simulink model "VB_RI_EKF_GNSS_INS25"  (R2023a)
settings: Solver=FixedStepAuto  StartTime=0  StopTime=200  FixedStep=0.01  RelTol=1e-3
InitFcn:
  | %resilient_initNavigation1216;
  | %init_param;
values from neighbouring files (symbols this model uses):
  C = zeros(n,m)    [utchol.m]
undefined symbols (not defined in the file or in its folder): dt, dtDelay, g0, gam0_rad, GNSSoutragetime, ISUS_flag, magnitude, p, P0, P0_RIEKF, param, pd0, pe0, phi0_rad, pn0, psi, psi0_rad, state_dim, vd0, ve0, vn0
libraries: simulink_extras x133, simulink x81, dspstat3 x81, sharedtransform x69, sharedTrackingLibrary x17, matrix_library x15, deeplib x6, dspfactors x4, aerolibconvert2 x4, aerolibtransform2 x4, dspsrcs4 x1
(part 13 of 32)

== system VB_RI_EKF_GNSS_INS25/ISUS_RIEKF3/Error State Kalman Filter M1/VB-Extended Kalman Filter M2 ==
  Q : Inport
  Enable1 : Inport  Port=2
  y1 : Inport  Port=3
  R1 : Inport  Port=4
  H : Inport  Port=5
  pk_1 : Inport  Port=6
  pk_2 : Inport  Port=7
  BlockOrdering : Constant  Value=true()  OutDataTypeStr=boolean
  Correct M1 : Subsystem  AncestorBlock=sharedTrackingLibrary/Extras/EKFCorrect  TreatAsAtomicUnit=on  SystemSampleTime=p.SampleTimes.MeasurementFcn(1)  mask(EKFCorrect){ProcessedMaskData=p}
      mask init: same as VB_RI_EKF_GNSS_INS25/ER EKF/Error State Kalman Filter/Extended Kalman Filter1/Correct1
      settings: LibrarySourceBlock=sharedTrackingLibrary/Extras/EKFCorrect
  Data Store Read : DataStoreRead  Commented=on  DataStoreName=P  IndexOptions=Index vector (dialog)  Indices=1  OutputSizes=1
  Data Store Read1 : DataStoreRead  Commented=on  DataStoreName=x  IndexOptions=Index vector (dialog)  Indices=1  OutputSizes=1
  DataStoreMemory - P : DataStoreMemory  DataStoreName=P  InitialValue=p.InitialCovariance  ShowAdditionalParam=off  OutDataTypeStr=p.DataType
  DataStoreMemory - x : DataStoreMemory  DataStoreName=x  InitialValue=p.InitialState  ShowAdditionalParam=off  OutDataTypeStr=p.DataType
  DataTypeConversion_Enable1 : DataTypeConversion  OutDataTypeStr=boolean  SaturateOnIntegerOverflow=off  RndMeth=Floor
  DataTypeConversion_Q : DataTypeConversion  OutDataTypeStr=p.DataType  SaturateOnIntegerOverflow=off  RndMeth=Floor
  DataTypeConversion_R1 : DataTypeConversion  OutDataTypeStr=p.DataType  SaturateOnIntegerOverflow=off  RndMeth=Floor
  DataTypeConversion_uMeas1 : DataTypeConversion  OutDataTypeStr=p.DataType  SaturateOnIntegerOverflow=off  RndMeth=Floor
  DataTypeConversion_uState : DataTypeConversion  OutDataTypeStr=p.DataType  SaturateOnIntegerOverflow=off  RndMeth=Floor
  DataTypeConversion_y1 : DataTypeConversion  OutDataTypeStr=p.DataType  SaturateOnIntegerOverflow=off  RndMeth=Floor
  MeasurementFcn1Inputs : Constant  Value=0  OutDataTypeStr=p.DataType  SampleTime=p.SampleTimes.MeasurementFcn(1)
  Output : Subsystem  TreatAsAtomicUnit=on  SystemSampleTime=p.SampleTimes.Output
  Predict : Subsystem  TreatAsAtomicUnit=on  SystemSampleTime=p.SampleTimes.StateTransitionFcn  mask(EKFPredict){ProcessedMaskData=p}
      mask init: same as VB_RI_EKF_GNSS_INS25/ER EKF/Error State Kalman Filter/Extended Kalman Filter1/Predict
  StateTransitionFcnInputs : Constant  Value=0  OutDataTypeStr=p.DataType  SampleTime=p.SampleTimes.StateTransitionFcn
  checkMeasurementFcn1Signals : S-Function  FunctionName=ekfukfCheckSignals  Parameters=signalCheck.BlockPath, signalCheck.MeasurementFcn{1}.PortNames, signalCheck.MeasurementFcn{1}.SampleTime, signalCheck.DataType, signalCheck.MeasurementFcn{1}.PortDimensions, 1, signalCheck.MeasurementFcn{1}.HasAdditiveNoise  SFunctionDeploymentMode=off  EnableBusSupport=off
  checkStateTransitionFcnSignals : S-Function  FunctionName=ekfukfCheckSignals  Parameters=signalCheck.BlockPath, signalCheck.StateTransitionFcn.PortNames, signalCheck.StateTransitionFcn.SampleTime, signalCheck.DataType, signalCheck.StateTransitionFcn.PortDimensions, 0, signalCheck.StateTransitionFcn.HasAdditiveNoise  SFunctionDeploymentMode=off  EnableBusSupport=off
  innovation calculation : Subsystem  Commented=on
  xhat : Outport  VectorParamsAs1DForOutWhenUnconnected=off
  P : Outport  Port=2
  Sk : Outport  Port=3  VectorParamsAs1DForOutWhenUnconnected=off
  m_innov : Outport  Port=4  VectorParamsAs1DForOutWhenUnconnected=off
  wires:
  [AfterOutput] -> Predict/3(uBlockOrdering)
  Output/3(yBlockOrdering) -> [AfterOutput]
  [AfterCorrect] -> Output/1(uBlockOrdering)
  [FirstOperation] -> Correct M1/4(uBlockOrdering)
  BlockOrdering/1 -> [FirstOperation]
  DataTypeConversion_uMeas1/1 -> Correct M1/3(uMeas)
  DataTypeConversion_R1/1 -> Correct M1/2(R), innovation calculation/4(R)
  MeasurementFcn1Inputs/1 -> DataTypeConversion_uMeas1/1, checkMeasurementFcn1Signals/4
  DataTypeConversion_y1/1 -> innovation calculation/2(yMeas), Correct M1/1(yMeas)
  DataTypeConversion_uState/1 -> Predict/2(uState)
  StateTransitionFcnInputs/1 -> DataTypeConversion_uState/1, checkStateTransitionFcnSignals/2
  DataTypeConversion_Enable1/1 -> Correct M1/Enable
  Enable1/1 -> DataTypeConversion_Enable1/1, checkMeasurementFcn1Signals/1
  DataTypeConversion_Q/1 -> Predict/1(Q)
  Q/1 -> DataTypeConversion_Q/1, checkStateTransitionFcnSignals/1
  R1/1 -> DataTypeConversion_R1/1, checkMeasurementFcn1Signals/3
  y1/1 -> DataTypeConversion_y1/1, checkMeasurementFcn1Signals/2
  Output/1(x) -> xhat/1
  Correct M1/1(yBlockOrdering) -> [AfterCorrect]
  H/1 -> innovation calculation/5(H), Correct M1/5(H)
  pk_1/1 -> Correct M1/6(pk_1)
  Output/2(P) -> P/1
  Data Store Read/1 -> innovation calculation/1(Pk/k_1)
  Data Store Read1/1 -> innovation calculation/3(X)
  Correct M1/2(Sk) -> Sk/1
  Correct M1/3(m_innov) -> m_innov/1
  pk_2/1 -> Correct M1/7(P)

== system VB_RI_EKF_GNSS_INS25/ISUS_RIEKF3/Error State Kalman Filter M1/bak ==
  From1 : From  Commented=on  GotoTag=wxyz
  From11 : From  Commented=on  GotoTag=p_INS
  From14 : From  Commented=on  GotoTag=DCM_b_n
  From2 : From  Commented=on  GotoTag=fbxyz
  From3 : From  Commented=on  GotoTag=ZUPTenable
  From4 : From  Commented=on  GotoTag=v_INS
  From5 : From  Commented=on  GotoTag=fex
  From6 : From  Commented=on  GotoTag=DCM_b_n
  From9 : From  Commented=on  GotoTag=DCM_b_n
  Goto6 : Goto  Commented=on  GotoTag=ZUPTenable
  MATLAB Function1 : MATLAB Function  Commented=on  TreatAsAtomicUnit=on
  Memory1 : Memory  Commented=on
  RIEKF : MATLAB Function  Commented=on  TreatAsAtomicUnit=on
  Rate Transition2 : RateTransition  Commented=on  OutPortSampleTime=dt
  Scope10 : Scope  Commented=on  NumInputPorts=2
  Simulink Function - GPS Measurements1 : Subsystem  Commented=on  TreatAsAtomicUnit=on
  Simulink Function - GPS Measurements2 : Subsystem  Commented=on  TreatAsAtomicUnit=on
  Simulink Function - State Transition Jacobian : Subsystem  Commented=on  TreatAsAtomicUnit=on
  Unscented Kalman Filter1 : sharedTrackingLibrary/Unscented Kalman Filter  Commented=on  StateTransitionFcn=stateTransitionFcn_Dyn  HasAdditiveProcessNoise=Nonadditive  ProcessNoise=1  HasTimeVaryingProcessNoise=on  HasStateTransitionFcnExtraArgument=0  InitialState=zeros(18,1)  InitialStateCovariance=diag([1*ones(3,1);0.1*ones(3,1);0.001*ones(3,1);0.001*ones(6,1);0.1*ones(3,1)]);  Alpha=1e-2  Beta=2  Kappa=0  MeasurementFcn1=GPSMeasurementFcn_Dyn  HasMeasurementEnablePort1=on  HasAdditiveMeasurementNoise1=Nonadditive  MeasurementNoise1=1  HasTimeVaryingMeasurementNoise1=on  HasMeasurementFcnExtraArgument1=0  HasMeasurementWrapping1=off  MeasurementFcn2=DynamicMeasurementFcn_Dyn  HasMeasurementEnablePort2=on  HasAdditiveMeasurementNoise2=Nonadditive  MeasurementNoise2=1  HasTimeVaryingMeasurementNoise2=on  HasMeasurementFcnExtraArgument2=0  HasMeasurementWrapping2=off  MeasurementFcn3=myMeasurementFcn  HasMeasurementEnablePort3=off  HasAdditiveMeasurementNoise3=Additive  MeasurementNoise3=1  HasTimeVaryingMeasurementNoise3=off  HasMeasurementFcnExtraArgument3=0  HasMeasurementWrapping3=off  MeasurementFcn4=myMeasurementFcn  HasMeasurementEnablePort4=off  HasAdditiveMeasurementNoise4=Additive  MeasurementNoise4=1  HasTimeVaryingMeasurementNoise4=off  HasMeasurementFcnExtraArgument4=0  HasMeasurementWrapping4=off  MeasurementFcn5=myMeasurementFcn  HasMeasurementEnablePort5=off  HasAdditiveMeasurementNoise5=Additive  MeasurementNoise5=1  HasTimeVaryingMeasurementNoise5=off  HasMeasurementFcnExtraArgument5=0  HasMeasurementWrapping5=off  EnableMultirate=off  StateTransitionFcnSampleTime=1  MeasurementFcn1SampleTime=1  MeasurementFcn2SampleTime=1  MeasurementFcn3SampleTime=1  MeasurementFcn4SampleTime=1  MeasurementFcn5SampleTime=1  UseCurrentEstimator=on  OutputStateCovariance=on  DataType=single  SampleTime=0.01  NumberOfMeasurements=2
  Out1 : Outport
  wires:
  From14/1 -> Simulink Function - GPS Measurements1/1(DCM_b_n)
  From4/1 -> Simulink Function - State Transition Jacobian/2(vn)
  From9/1 -> Simulink Function - State Transition Jacobian/1(DCM_b_n)
  From11/1 -> Simulink Function - State Transition Jacobian/3(pn)
  From3/1 -> Rate Transition2/1
  MATLAB Function1/2(ZeroVelDetectFlagold) -> Scope10/2
  From6/1 -> MATLAB Function1/1(Cbn)
  From2/1 -> MATLAB Function1/3(fbxyz)
  From5/1 -> Memory1/1
  MATLAB Function1/1(ZeroVelDetectFlag) -> Goto6/1, Scope10/1
  From1/1 -> MATLAB Function1/2(wxyz)
  Rate Transition2/1 -> Out1/1
  Memory1/1 -> MATLAB Function1/4(fex)

== system VB_RI_EKF_GNSS_INS25/ISUS_RIEKF3/Error State Kalman Filter M2/Cal Q1 ==
  Constant : Constant  Value=dt  OutDataTypeStr=double
  MATLAB Function1 : MATLAB Function  TreatAsAtomicUnit=on
  Qd : Outport
  wires:
  Constant/1 -> MATLAB Function1/1(dt)
  MATLAB Function1/1(Q) -> Qd/1

== system VB_RI_EKF_GNSS_INS25/ISUS_RIEKF3/Error State Kalman Filter M2/Extended Kalman Filter M1 ==
  Q : Inport
  Enable1 : Inport  Port=2
  y1 : Inport  Port=3
  R1 : Inport  Port=4
  H : Inport  Port=5
  pk_1 : Inport  Port=6
  beta_2 : Inport  Port=7
  BlockOrdering : Constant  Value=true()  OutDataTypeStr=boolean
  Correct M1 : Subsystem  AncestorBlock=sharedTrackingLibrary/Extras/EKFCorrect  TreatAsAtomicUnit=on  SystemSampleTime=p.SampleTimes.MeasurementFcn(1)  mask(EKFCorrect){ProcessedMaskData=p}
      mask init: same as VB_RI_EKF_GNSS_INS25/ER EKF/Error State Kalman Filter/Extended Kalman Filter1/Correct1
      settings: LibrarySourceBlock=sharedTrackingLibrary/Extras/EKFCorrect
  DataStoreMemory - P : DataStoreMemory  DataStoreName=P  InitialValue=p.InitialCovariance  ShowAdditionalParam=off  OutDataTypeStr=p.DataType
  DataStoreMemory - x : DataStoreMemory  DataStoreName=x  InitialValue=p.InitialState  ShowAdditionalParam=off  OutDataTypeStr=p.DataType
  DataTypeConversion_Enable1 : DataTypeConversion  OutDataTypeStr=boolean  SaturateOnIntegerOverflow=off  RndMeth=Floor
  DataTypeConversion_Q : DataTypeConversion  OutDataTypeStr=p.DataType  SaturateOnIntegerOverflow=off  RndMeth=Floor
  DataTypeConversion_R1 : DataTypeConversion  OutDataTypeStr=p.DataType  SaturateOnIntegerOverflow=off  RndMeth=Floor
  DataTypeConversion_uMeas1 : DataTypeConversion  OutDataTypeStr=p.DataType  SaturateOnIntegerOverflow=off  RndMeth=Floor
  DataTypeConversion_uState : DataTypeConversion  OutDataTypeStr=p.DataType  SaturateOnIntegerOverflow=off  RndMeth=Floor
  DataTypeConversion_y1 : DataTypeConversion  OutDataTypeStr=p.DataType  SaturateOnIntegerOverflow=off  RndMeth=Floor
  MeasurementFcn1Inputs : Constant  Value=0  OutDataTypeStr=p.DataType  SampleTime=p.SampleTimes.MeasurementFcn(1)
  Output : Subsystem  TreatAsAtomicUnit=on  SystemSampleTime=p.SampleTimes.Output
  Predict : Subsystem  TreatAsAtomicUnit=on  SystemSampleTime=p.SampleTimes.StateTransitionFcn  mask(EKFPredict){ProcessedMaskData=p}
      mask init: same as VB_RI_EKF_GNSS_INS25/ER EKF/Error State Kalman Filter/Extended Kalman Filter1/Predict
  StateTransitionFcnInputs : Constant  Value=0  OutDataTypeStr=p.DataType  SampleTime=p.SampleTimes.StateTransitionFcn
  checkMeasurementFcn1Signals : S-Function  FunctionName=ekfukfCheckSignals  Parameters=signalCheck.BlockPath, signalCheck.MeasurementFcn{1}.PortNames, signalCheck.MeasurementFcn{1}.SampleTime, signalCheck.DataType, signalCheck.MeasurementFcn{1}.PortDimensions, 1, signalCheck.MeasurementFcn{1}.HasAdditiveNoise  SFunctionDeploymentMode=off  EnableBusSupport=off
  checkStateTransitionFcnSignals : S-Function  FunctionName=ekfukfCheckSignals  Parameters=signalCheck.BlockPath, signalCheck.StateTransitionFcn.PortNames, signalCheck.StateTransitionFcn.SampleTime, signalCheck.DataType, signalCheck.StateTransitionFcn.PortDimensions, 0, signalCheck.StateTransitionFcn.HasAdditiveNoise  SFunctionDeploymentMode=off  EnableBusSupport=off
  xhat : Outport  VectorParamsAs1DForOutWhenUnconnected=off
  P : Outport  Port=2
  Sk : Outport  Port=3  VectorParamsAs1DForOutWhenUnconnected=off
  m_innov : Outport  Port=4  VectorParamsAs1DForOutWhenUnconnected=off
  beta2 : Outport  Port=5  VectorParamsAs1DForOutWhenUnconnected=off
  wires:
  [AfterOutput] -> Predict/3(uBlockOrdering)
  Output/3(yBlockOrdering) -> [AfterOutput]
  [AfterCorrect] -> Output/1(uBlockOrdering)
  [FirstOperation] -> Correct M1/4(uBlockOrdering)
  BlockOrdering/1 -> [FirstOperation]
  DataTypeConversion_uMeas1/1 -> Correct M1/3(uMeas)
  DataTypeConversion_R1/1 -> Correct M1/2(R)
  MeasurementFcn1Inputs/1 -> DataTypeConversion_uMeas1/1, checkMeasurementFcn1Signals/4
  DataTypeConversion_y1/1 -> Correct M1/1(yMeas)
  DataTypeConversion_uState/1 -> Predict/2(uState)
  StateTransitionFcnInputs/1 -> DataTypeConversion_uState/1, checkStateTransitionFcnSignals/2
  DataTypeConversion_Enable1/1 -> Correct M1/Enable
  Enable1/1 -> DataTypeConversion_Enable1/1, checkMeasurementFcn1Signals/1
  DataTypeConversion_Q/1 -> Predict/1(Q)
  Q/1 -> DataTypeConversion_Q/1, checkStateTransitionFcnSignals/1
  R1/1 -> DataTypeConversion_R1/1, checkMeasurementFcn1Signals/3
  y1/1 -> DataTypeConversion_y1/1, checkMeasurementFcn1Signals/2
  Output/1(x) -> xhat/1
  Correct M1/1(yBlockOrdering) -> [AfterCorrect]
  Correct M1/2(Sk) -> Sk/1
  Correct M1/3(m_innov) -> m_innov/1
  H/1 -> Correct M1/5(H)
  pk_1/1 -> Correct M1/6(pk_1)
  Output/2(P) -> P/1
  Correct M1/4(beta2) -> beta2/1
  beta_2/1 -> Correct M1/7(beta_2)

== system VB_RI_EKF_GNSS_INS25/ISUS_RIEKF3/Error State Kalman Filter M2/Simulink Function - GPS Measurements ==
  Rbn : Inport
  vn : Inport  Port=2
  pn : Inport  Port=3
  GPSMeasurementFcn_RIEKF : TriggerPort  TriggerType=function-call  IsSimulinkFunction=on  FunctionName=GPSMeasurementFcn_RIEKF  FunctionVisibility=scoped  VariantControl=Variant
  Add : Sum
  Data Type Conversion1 : DataTypeConversion  OutDataTypeStr=single  SaturateOnIntegerOverflow=off  RndMeth=Floor
  MATLAB Function : MATLAB Function  TreatAsAtomicUnit=on
  MATLAB Function1 : MATLAB Function  Commented=on  TreatAsAtomicUnit=on
  Product : Product  Multiplication=Matrix(*)
  pn1 : InportShadow  Port=3
  vn1 : InportShadow  Port=2
  x : ArgIn  DisableCoverage=on  OutDataTypeStr=single  PortDimensions=state_dim  ArgumentName=x
  v : ArgIn  DisableCoverage=on  Port=2  OutDataTypeStr=single  PortDimensions=6  ArgumentName=v
  y : ArgOut  DisableCoverage=on  OutDataTypeStr=single  PortDimensions=6  ArgumentName=y
  H : Outport
  wires:
  MATLAB Function/1(H) -> Data Type Conversion1/1
  Product/1 -> Add/1
  Add/1 -> y/1
  vn/1 -> MATLAB Function/1(vn)
  Rbn/1 -> MATLAB Function1/1(Rbn)
  vn1/1 -> MATLAB Function1/2(vn)
  pn1/1 -> MATLAB Function1/3(pn)
  x/1 -> Product/2
  v/1 -> Add/2
  pn/1 -> MATLAB Function/2(pn)
  Data Type Conversion1/1 -> H/1, Product/1

== system VB_RI_EKF_GNSS_INS25/ISUS_RIEKF3/Error State Kalman Filter M2/Simulink Function - GPS Measurements1 ==
  vn : Inport
  pn : Inport  Port=2
  BaroMeasurementFcn_RIEKF : TriggerPort  TriggerType=function-call  IsSimulinkFunction=on  FunctionName=BaroMeasurementFcn_RIEKF  VariantControl=Variant
  Add : Sum
  Data Type Conversion1 : DataTypeConversion  OutDataTypeStr=single  SaturateOnIntegerOverflow=off  RndMeth=Floor
  MATLAB Function : MATLAB Function  TreatAsAtomicUnit=on
  Product : Product  Multiplication=Matrix(*)
  x : ArgIn  DisableCoverage=on  OutDataTypeStr=single  PortDimensions=state_dim  ArgumentName=x
  v : ArgIn  DisableCoverage=on  Port=2  OutDataTypeStr=single  ArgumentName=v
  y : ArgOut  DisableCoverage=on  OutDataTypeStr=single  ArgumentName=y
  wires:
  MATLAB Function/1(H_baro) -> Data Type Conversion1/1
  Product/1 -> Add/1
  Add/1 -> y/1
  vn/1 -> MATLAB Function/1(vn)
  x/1 -> Product/2
  v/1 -> Add/2
  pn/1 -> MATLAB Function/2(pn)
  Data Type Conversion1/1 -> Product/1

== system VB_RI_EKF_GNSS_INS25/ISUS_RIEKF3/Error State Kalman Filter M2/Simulink Function - GPS Measurements2 ==
  Rbn : Inport
  Magn : Inport  Port=2
  xstate : Inport  Port=3
  MagnMeasurementFcn_RIEKF : TriggerPort  TriggerType=function-call  IsSimulinkFunction=on  FunctionName=MagnMeasurementFcn_RIEKF  VariantControl=Variant
  Add : Sum
  Data Type Conversion1 : DataTypeConversion  OutDataTypeStr=single  SaturateOnIntegerOverflow=off  RndMeth=Floor
  MATLAB Function : MATLAB Function  TreatAsAtomicUnit=on
  Product : Product  Multiplication=Matrix(*)
  Selector : Selector  InputPortWidth=state_dim  IndexOptions=Index vector (dialog)  Indices=[1 2 3]  OutputSizes=1
  x : ArgIn  DisableCoverage=on  OutDataTypeStr=single  PortDimensions=state_dim  ArgumentName=x
  v : ArgIn  DisableCoverage=on  Port=2  OutDataTypeStr=single  PortDimensions=3  ArgumentName=v
  y : ArgOut  DisableCoverage=on  OutDataTypeStr=single  PortDimensions=3  ArgumentName=y
  wires:
  MATLAB Function/1(H) -> Data Type Conversion1/1
  Product/1 -> Add/1
  Add/1 -> y/1
  Magn/1 -> MATLAB Function/2(Magn)
  x/1 -> Product/2
  v/1 -> Add/2
  Data Type Conversion1/1 -> Product/1
  Rbn/1 -> MATLAB Function/1(Rbn)
  xstate/1 -> Selector/1
  Selector/1 -> MATLAB Function/3(dtheta)

== system VB_RI_EKF_GNSS_INS25/ISUS_RIEKF3/Error State Kalman Filter M2/Simulink Function - GPS Measurements3 ==
  Rbn : Inport
  vn : Inport  Port=2
  Rab : Inport  Port=3
  vel_wind_NED : Inport  Port=4
  AirspeedMeasurementFcn_RIEKF : TriggerPort  TriggerType=function-call  IsSimulinkFunction=on  FunctionName=AirspeedMeasurementFcn_RIEKF  VariantControl=Variant
  Add : Sum
  Data Type Conversion1 : DataTypeConversion  OutDataTypeStr=single  SaturateOnIntegerOverflow=off  RndMeth=Floor
  MATLAB Function : MATLAB Function  TreatAsAtomicUnit=on
  Product : Product  Multiplication=Matrix(*)
  x : ArgIn  DisableCoverage=on  OutDataTypeStr=single  PortDimensions=state_dim  ArgumentName=x
  v : ArgIn  DisableCoverage=on  Port=2  OutDataTypeStr=single  PortDimensions=3  ArgumentName=v
  y : ArgOut  DisableCoverage=on  OutDataTypeStr=single  PortDimensions=3  ArgumentName=y
  wires:
  MATLAB Function/1(H) -> Data Type Conversion1/1
  Product/1 -> Add/1
  Add/1 -> y/1
  x/1 -> Product/2
  v/1 -> Add/2
  Data Type Conversion1/1 -> Product/1
  Rbn/1 -> MATLAB Function/1(Rbn)
  vn/1 -> MATLAB Function/3(vn)
  Rab/1 -> MATLAB Function/2(Rab)
  vel_wind_NED/1 -> MATLAB Function/4(v_wind)

== system VB_RI_EKF_GNSS_INS25/ISUS_RIEKF3/Error State Kalman Filter M2/Simulink Function - State Transition ==
  DCM_b_n : Inport
  vn : Inport  Port=2  PortDimensions=[3,1]
  pn : Inport  Port=3  PortDimensions=[3,1]
  stateTransitionFcn_RIEKF : TriggerPort  TriggerType=function-call  IsSimulinkFunction=on  FunctionName=stateTransitionFcn_RIEKF  FunctionVisibility=scoped  VariantControl=Variant
  Add : Sum
  Cal Phi : Subsystem
  Constant : Constant  Value=dt  OutDataTypeStr=single
  Data Type Conversion1 : DataTypeConversion  OutDataTypeStr=single  SaturateOnIntegerOverflow=off  RndMeth=Floor
  Data Type Conversion6 : DataTypeConversion  OutDataTypeStr=single  SaturateOnIntegerOverflow=off  RndMeth=Floor
  MATLAB Function : MATLAB Function  TreatAsAtomicUnit=on
  Product1 : Product  Multiplication=Matrix(*)
  Product2 : Product  Multiplication=Matrix(*)
  x : ArgIn  DisableCoverage=on  OutDataTypeStr=single  PortDimensions=state_dim  ArgumentName=x
  w : ArgIn  Port=2  OutDataTypeStr=single  PortDimensions=cov_dim  ArgumentName=w
  xNext : ArgOut  DisableCoverage=on  OutDataTypeStr=single  PortDimensions=state_dim  ArgumentName=xNext
  wires:
  x/1 -> Product2/2
  Product2/1 -> Data Type Conversion6/1
  MATLAB Function/1(G) -> Product1/1
  w/1 -> Product1/2
  Product1/1 -> Data Type Conversion1/1
  Add/1 -> xNext/1
  [DCM_b_n] -> MATLAB Function/1(Rbn)
  Constant/1 -> MATLAB Function/4(dt)
  DCM_b_n/1 -> [DCM_b_n]
  Cal Phi/1(Phi) -> Product2/1
  Data Type Conversion6/1 -> Add/2
  [DCM_b_n] -> Cal Phi/1(Rbn)
  vn/1 -> MATLAB Function/2(vn), Cal Phi/2(vn)
  pn/1 -> MATLAB Function/3(pn), Cal Phi/3(pn)
  Data Type Conversion1/1 -> Add/1

== system VB_RI_EKF_GNSS_INS25/ISUS_RIEKF3/Error State Kalman Filter M2/Simulink Function - State Transition1 ==
  DCM_b_n : Inport
  vn : Inport  Port=2  PortDimensions=[3,1]
  pn : Inport  Port=3  PortDimensions=[3,1]
  stateFcn_RIEKFJacobian : TriggerPort  TriggerType=function-call  IsSimulinkFunction=on  FunctionName=stateFcn_RIEKFJacobian  FunctionVisibility=scoped  VariantControl=Variant
  Cal Phi : Subsystem
  Constant : Constant  Value=dt  OutDataTypeStr=single
  Data Type Conversion1 : DataTypeConversion  OutDataTypeStr=single  SaturateOnIntegerOverflow=off  RndMeth=Floor
  Data Type Conversion6 : DataTypeConversion  OutDataTypeStr=single  SaturateOnIntegerOverflow=off  RndMeth=Floor
  MATLAB Function : MATLAB Function  TreatAsAtomicUnit=on
  Terminator : Terminator
  Terminator1 : Terminator
  x : ArgIn  DisableCoverage=on  OutDataTypeStr=single  PortDimensions=state_dim  ArgumentName=x
  w : ArgIn  Port=2  OutDataTypeStr=single  PortDimensions=cov_dim  ArgumentName=w
  A : ArgOut  DisableCoverage=on  OutDataTypeStr=single  PortDimensions=[state_dim,state_dim]  ArgumentName=A
  G : ArgOut  Port=2  OutDataTypeStr=single  PortDimensions=[15,12]  ArgumentName=G
  wires:
  pn/1 -> Cal Phi/3(pn), MATLAB Function/3(pn)
  vn/1 -> Cal Phi/2(vn), MATLAB Function/2(vn)
  [DCM_b_n] -> Cal Phi/1(Rbn)
  DCM_b_n/1 -> [DCM_b_n]
  Constant/1 -> MATLAB Function/4(dt)
  [DCM_b_n] -> MATLAB Function/1(Rbn)
  w/1 -> Terminator/1
  x/1 -> Terminator1/1
  MATLAB Function/1(G) -> Data Type Conversion6/1
  Cal Phi/1(Phi) -> Data Type Conversion1/1
  Data Type Conversion6/1 -> G/1
  Data Type Conversion1/1 -> A/1

== system VB_RI_EKF_GNSS_INS25/ISUS_RIEKF3/Error State Kalman Filter M2/Subsystem ==
  data : Inport
  Detect Change : simulink/Logic and Bit Operations/Detect Change  vinit=0  InputProcessing=Columns as channels (frame based)  OutDataTypeStr=boolean
  Selector : Selector  InputPortWidth=3  IndexOptions=Index vector (dialog)  Indices=[3]  OutputSizes=1
  Zero-Order Hold : ZeroOrderHold  SampleTime=0.2
  Zero-Order Hold1 : ZeroOrderHold  SampleTime=0.01
  flag : Outport
  wires:
  Zero-Order Hold1/1 -> Detect Change/1
  Detect Change/1 -> flag/1
  Selector/1 -> Zero-Order Hold1/1
  data/1 -> Zero-Order Hold/1
  Zero-Order Hold/1 -> Selector/1

== system VB_RI_EKF_GNSS_INS25/ISUS_RIEKF3/Error State Kalman Filter M2/Subsystem1 ==
  v_I : Inport
  v_G : Inport  Port=2
  p_I : Inport  Port=3
  p_G : Inport  Port=4
  Enable : EnablePort
  Add1 : Sum  Inputs=+-
  Add2 : Sum  Inputs=+-
  Data Type Conversion : DataTypeConversion  OutDataTypeStr=single  SaturateOnIntegerOverflow=off  RndMeth=Floor
  Data Type Conversion2 : DataTypeConversion  OutDataTypeStr=single  SaturateOnIntegerOverflow=off  RndMeth=Floor
  Gain : Gain  Gain=-1
  Mux2 : Mux  Inputs=2
  dv/dp : Outport
  wires:
  Mux2/1 -> Gain/1
  Data Type Conversion2/1 -> Mux2/1
  v_G/1 -> Add2/2
  Data Type Conversion/1 -> Mux2/2
  p_I/1 -> Add1/1
  Add1/1 -> Data Type Conversion/1
  Add2/1 -> Data Type Conversion2/1
  v_I/1 -> Add2/1
  Gain/1 -> dv/dp/1
  p_G/1 -> Add1/2

== system VB_RI_EKF_GNSS_INS25/ISUS_RIEKF3/Error State Kalman Filter M2/Subsystem3 ==
  data : Inport
  Detect Change : simulink/Logic and Bit Operations/Detect Change  vinit=0  InputProcessing=Columns as channels (frame based)  OutDataTypeStr=boolean
  From Workspace1 : FromWorkspace  Commented=on  VariableName=[All.t',All.vn]
  From Workspace2 : FromWorkspace  VariableName=[time(1:(end-1)),FCS1.data_hf_st.lat(1:(end-1))]
  Selector : Selector  InputPortWidth=3  IndexOptions=Index vector (dialog)  Indices=[3]  OutputSizes=1
  flag : Outport
  wires:
  Detect Change/1 -> flag/1
  data/1 -> Selector/1
  From Workspace2/1 -> Detect Change/1  "lat"

== system VB_RI_EKF_GNSS_INS25/ISUS_RIEKF3/Error State Kalman Filter M2/bak ==
  From1 : From  Commented=on  GotoTag=wxyz
  From11 : From  Commented=on  GotoTag=p_INS
  From14 : From  Commented=on  GotoTag=DCM_b_n
  From2 : From  Commented=on  GotoTag=fbxyz
  From3 : From  Commented=on  GotoTag=ZUPTenable
  From4 : From  Commented=on  GotoTag=v_INS
  From5 : From  Commented=on  GotoTag=fex
  From6 : From  Commented=on  GotoTag=DCM_b_n
  From9 : From  Commented=on  GotoTag=DCM_b_n
  Goto6 : Goto  Commented=on  GotoTag=ZUPTenable
  MATLAB Function1 : MATLAB Function  Commented=on  TreatAsAtomicUnit=on
  Memory1 : Memory  Commented=on
  RIEKF : MATLAB Function  Commented=on  TreatAsAtomicUnit=on
  Rate Transition2 : RateTransition  Commented=on  OutPortSampleTime=dt
  Scope10 : Scope  Commented=on  NumInputPorts=2
  Simulink Function - GPS Measurements1 : Subsystem  Commented=on  TreatAsAtomicUnit=on
  Simulink Function - GPS Measurements2 : Subsystem  Commented=on  TreatAsAtomicUnit=on
  Simulink Function - State Transition Jacobian : Subsystem  Commented=on  TreatAsAtomicUnit=on
  Unscented Kalman Filter1 : sharedTrackingLibrary/Unscented Kalman Filter  Commented=on  StateTransitionFcn=stateTransitionFcn_Dyn  HasAdditiveProcessNoise=Nonadditive  ProcessNoise=1  HasTimeVaryingProcessNoise=on  HasStateTransitionFcnExtraArgument=0  InitialState=zeros(18,1)  InitialStateCovariance=diag([1*ones(3,1);0.1*ones(3,1);0.001*ones(3,1);0.001*ones(6,1);0.1*ones(3,1)]);  Alpha=1e-2  Beta=2  Kappa=0  MeasurementFcn1=GPSMeasurementFcn_Dyn  HasMeasurementEnablePort1=on  HasAdditiveMeasurementNoise1=Nonadditive  MeasurementNoise1=1  HasTimeVaryingMeasurementNoise1=on  HasMeasurementFcnExtraArgument1=0  HasMeasurementWrapping1=off  MeasurementFcn2=DynamicMeasurementFcn_Dyn  HasMeasurementEnablePort2=on  HasAdditiveMeasurementNoise2=Nonadditive  MeasurementNoise2=1  HasTimeVaryingMeasurementNoise2=on  HasMeasurementFcnExtraArgument2=0  HasMeasurementWrapping2=off  MeasurementFcn3=myMeasurementFcn  HasMeasurementEnablePort3=off  HasAdditiveMeasurementNoise3=Additive  MeasurementNoise3=1  HasTimeVaryingMeasurementNoise3=off  HasMeasurementFcnExtraArgument3=0  HasMeasurementWrapping3=off  MeasurementFcn4=myMeasurementFcn  HasMeasurementEnablePort4=off  HasAdditiveMeasurementNoise4=Additive  MeasurementNoise4=1  HasTimeVaryingMeasurementNoise4=off  HasMeasurementFcnExtraArgument4=0  HasMeasurementWrapping4=off  MeasurementFcn5=myMeasurementFcn  HasMeasurementEnablePort5=off  HasAdditiveMeasurementNoise5=Additive  MeasurementNoise5=1  HasTimeVaryingMeasurementNoise5=off  HasMeasurementFcnExtraArgument5=0  HasMeasurementWrapping5=off  EnableMultirate=off  StateTransitionFcnSampleTime=1  MeasurementFcn1SampleTime=1  MeasurementFcn2SampleTime=1  MeasurementFcn3SampleTime=1  MeasurementFcn4SampleTime=1  MeasurementFcn5SampleTime=1  UseCurrentEstimator=on  OutputStateCovariance=on  DataType=single  SampleTime=0.01  NumberOfMeasurements=2
  Out1 : Outport
  wires:
  Memory1/1 -> MATLAB Function1/4(fex)
  Rate Transition2/1 -> Out1/1
  From1/1 -> MATLAB Function1/2(wxyz)
  MATLAB Function1/1(ZeroVelDetectFlag) -> Scope10/1, Goto6/1
  From5/1 -> Memory1/1
  From2/1 -> MATLAB Function1/3(fbxyz)
  From6/1 -> MATLAB Function1/1(Cbn)
  MATLAB Function1/2(ZeroVelDetectFlagold) -> Scope10/2
  From3/1 -> Rate Transition2/1
  From11/1 -> Simulink Function - State Transition Jacobian/3(pn)
  From9/1 -> Simulink Function - State Transition Jacobian/1(DCM_b_n)
  From4/1 -> Simulink Function - State Transition Jacobian/2(vn)
  From14/1 -> Simulink Function - GPS Measurements1/1(DCM_b_n)

== system VB_RI_EKF_GNSS_INS25/ISUS_RIEKF3/Error State Kalman Filter M3/Cal Q1 ==
  Constant : Constant  Value=dt  OutDataTypeStr=double
  MATLAB Function1 : MATLAB Function  TreatAsAtomicUnit=on
  Qd : Outport
  wires:
  MATLAB Function1/1(Q) -> Qd/1
  Constant/1 -> MATLAB Function1/1(dt)

== system VB_RI_EKF_GNSS_INS25/ISUS_RIEKF3/Error State Kalman Filter M3/Extended Kalman Filter M1 ==
  Q : Inport
  Enable1 : Inport  Port=2
  y1 : Inport  Port=3
  R1 : Inport  Port=4
  H : Inport  Port=5
  pk_1 : Inport  Port=6
  beta_3 : Inport  Port=7
  BlockOrdering : Constant  Value=true()  OutDataTypeStr=boolean
  Correct M1 : Subsystem  AncestorBlock=sharedTrackingLibrary/Extras/EKFCorrect  TreatAsAtomicUnit=on  SystemSampleTime=p.SampleTimes.MeasurementFcn(1)  mask(EKFCorrect){ProcessedMaskData=p}
      mask init: same as VB_RI_EKF_GNSS_INS25/ER EKF/Error State Kalman Filter/Extended Kalman Filter1/Correct1
      settings: LibrarySourceBlock=sharedTrackingLibrary/Extras/EKFCorrect
  DataStoreMemory - P : DataStoreMemory  DataStoreName=P  InitialValue=p.InitialCovariance  ShowAdditionalParam=off  OutDataTypeStr=p.DataType
  DataStoreMemory - x : DataStoreMemory  DataStoreName=x  InitialValue=p.InitialState  ShowAdditionalParam=off  OutDataTypeStr=p.DataType
  DataTypeConversion_Enable1 : DataTypeConversion  OutDataTypeStr=boolean  SaturateOnIntegerOverflow=off  RndMeth=Floor
  DataTypeConversion_Q : DataTypeConversion  OutDataTypeStr=p.DataType  SaturateOnIntegerOverflow=off  RndMeth=Floor
  DataTypeConversion_R1 : DataTypeConversion  OutDataTypeStr=p.DataType  SaturateOnIntegerOverflow=off  RndMeth=Floor
  DataTypeConversion_uMeas1 : DataTypeConversion  OutDataTypeStr=p.DataType  SaturateOnIntegerOverflow=off  RndMeth=Floor
  DataTypeConversion_uState : DataTypeConversion  OutDataTypeStr=p.DataType  SaturateOnIntegerOverflow=off  RndMeth=Floor
  DataTypeConversion_y1 : DataTypeConversion  OutDataTypeStr=p.DataType  SaturateOnIntegerOverflow=off  RndMeth=Floor
  MeasurementFcn1Inputs : Constant  Value=0  OutDataTypeStr=p.DataType  SampleTime=p.SampleTimes.MeasurementFcn(1)
  Output : Subsystem  TreatAsAtomicUnit=on  SystemSampleTime=p.SampleTimes.Output
  Predict : Subsystem  TreatAsAtomicUnit=on  SystemSampleTime=p.SampleTimes.StateTransitionFcn  mask(EKFPredict){ProcessedMaskData=p}
      mask init: same as VB_RI_EKF_GNSS_INS25/ER EKF/Error State Kalman Filter/Extended Kalman Filter1/Predict
  StateTransitionFcnInputs : Constant  Value=0  OutDataTypeStr=p.DataType  SampleTime=p.SampleTimes.StateTransitionFcn
  checkMeasurementFcn1Signals : S-Function  FunctionName=ekfukfCheckSignals  Parameters=signalCheck.BlockPath, signalCheck.MeasurementFcn{1}.PortNames, signalCheck.MeasurementFcn{1}.SampleTime, signalCheck.DataType, signalCheck.MeasurementFcn{1}.PortDimensions, 1, signalCheck.MeasurementFcn{1}.HasAdditiveNoise  SFunctionDeploymentMode=off  EnableBusSupport=off
  checkStateTransitionFcnSignals : S-Function  FunctionName=ekfukfCheckSignals  Parameters=signalCheck.BlockPath, signalCheck.StateTransitionFcn.PortNames, signalCheck.StateTransitionFcn.SampleTime, signalCheck.DataType, signalCheck.StateTransitionFcn.PortDimensions, 0, signalCheck.StateTransitionFcn.HasAdditiveNoise  SFunctionDeploymentMode=off  EnableBusSupport=off
  xhat : Outport  VectorParamsAs1DForOutWhenUnconnected=off
  P : Outport  Port=2
  Sk : Outport  Port=3  VectorParamsAs1DForOutWhenUnconnected=off
  m_innov : Outport  Port=4  VectorParamsAs1DForOutWhenUnconnected=off
  beta3 : Outport  Port=5  VectorParamsAs1DForOutWhenUnconnected=off
  wires:
  Output/2(P) -> P/1
  pk_1/1 -> Correct M1/6(pk_1)
  H/1 -> Correct M1/5(H)
  Correct M1/3(m_innov) -> m_innov/1
  Correct M1/2(Sk) -> Sk/1
  Correct M1/1(yBlockOrdering) -> [AfterCorrect]
  Output/1(x) -> xhat/1
  y1/1 -> checkMeasurementFcn1Signals/2, DataTypeConversion_y1/1
  R1/1 -> checkMeasurementFcn1Signals/3, DataTypeConversion_R1/1
  Q/1 -> checkStateTransitionFcnSignals/1, DataTypeConversion_Q/1
  DataTypeConversion_Q/1 -> Predict/1(Q)
  Enable1/1 -> checkMeasurementFcn1Signals/1, DataTypeConversion_Enable1/1
  DataTypeConversion_Enable1/1 -> Correct M1/Enable
  StateTransitionFcnInputs/1 -> checkStateTransitionFcnSignals/2, DataTypeConversion_uState/1
  DataTypeConversion_uState/1 -> Predict/2(uState)
  DataTypeConversion_y1/1 -> Correct M1/1(yMeas)
  MeasurementFcn1Inputs/1 -> checkMeasurementFcn1Signals/4, DataTypeConversion_uMeas1/1
  DataTypeConversion_R1/1 -> Correct M1/2(R)
  DataTypeConversion_uMeas1/1 -> Correct M1/3(uMeas)
  BlockOrdering/1 -> [FirstOperation]
  [FirstOperation] -> Correct M1/4(uBlockOrdering)
  [AfterCorrect] -> Output/1(uBlockOrdering)
  Output/3(yBlockOrdering) -> [AfterOutput]
  [AfterOutput] -> Predict/3(uBlockOrdering)
  Correct M1/4(beta3) -> beta3/1
  beta_3/1 -> Correct M1/7(beta_3)

== system VB_RI_EKF_GNSS_INS25/ISUS_RIEKF3/Error State Kalman Filter M3/Simulink Function - GPS Measurements ==
  Rbn : Inport
  vn : Inport  Port=2
  pn : Inport  Port=3
  GPSMeasurementFcn_RIEKF : TriggerPort  TriggerType=function-call  IsSimulinkFunction=on  FunctionName=GPSMeasurementFcn_RIEKF  FunctionVisibility=scoped  VariantControl=Variant
  Add : Sum
  Data Type Conversion1 : DataTypeConversion  OutDataTypeStr=single  SaturateOnIntegerOverflow=off  RndMeth=Floor
  MATLAB Function : MATLAB Function  TreatAsAtomicUnit=on
  MATLAB Function1 : MATLAB Function  Commented=on  TreatAsAtomicUnit=on
  Product : Product  Multiplication=Matrix(*)
  pn1 : InportShadow  Port=3
  vn1 : InportShadow  Port=2
  x : ArgIn  DisableCoverage=on  OutDataTypeStr=single  PortDimensions=state_dim  ArgumentName=x
  v : ArgIn  DisableCoverage=on  Port=2  OutDataTypeStr=single  PortDimensions=6  ArgumentName=v
  y : ArgOut  DisableCoverage=on  OutDataTypeStr=single  PortDimensions=6  ArgumentName=y
  H : Outport
  wires:
  Data Type Conversion1/1 -> Product/1, H/1
  pn/1 -> MATLAB Function/2(pn)
  v/1 -> Add/2
  x/1 -> Product/2
  pn1/1 -> MATLAB Function1/3(pn)
  vn1/1 -> MATLAB Function1/2(vn)
  Rbn/1 -> MATLAB Function1/1(Rbn)
  vn/1 -> MATLAB Function/1(vn)
  Add/1 -> y/1
  Product/1 -> Add/1
  MATLAB Function/1(H) -> Data Type Conversion1/1

== system VB_RI_EKF_GNSS_INS25/ISUS_RIEKF3/Error State Kalman Filter M3/Simulink Function - GPS Measurements1 ==
  vn : Inport
  pn : Inport  Port=2
  BaroMeasurementFcn_RIEKF : TriggerPort  TriggerType=function-call  IsSimulinkFunction=on  FunctionName=BaroMeasurementFcn_RIEKF  VariantControl=Variant
  Add : Sum
  Data Type Conversion1 : DataTypeConversion  OutDataTypeStr=single  SaturateOnIntegerOverflow=off  RndMeth=Floor
  MATLAB Function : MATLAB Function  TreatAsAtomicUnit=on
  Product : Product  Multiplication=Matrix(*)
  x : ArgIn  DisableCoverage=on  OutDataTypeStr=single  PortDimensions=state_dim  ArgumentName=x
  v : ArgIn  DisableCoverage=on  Port=2  OutDataTypeStr=single  ArgumentName=v
  y : ArgOut  DisableCoverage=on  OutDataTypeStr=single  ArgumentName=y
  wires:
  Data Type Conversion1/1 -> Product/1
  pn/1 -> MATLAB Function/2(pn)
  v/1 -> Add/2
  x/1 -> Product/2
  vn/1 -> MATLAB Function/1(vn)
  Add/1 -> y/1
  Product/1 -> Add/1
  MATLAB Function/1(H_baro) -> Data Type Conversion1/1

== system VB_RI_EKF_GNSS_INS25/ISUS_RIEKF3/Error State Kalman Filter M3/Simulink Function - GPS Measurements2 ==
  Rbn : Inport
  Magn : Inport  Port=2
  xstate : Inport  Port=3
  MagnMeasurementFcn_RIEKF : TriggerPort  TriggerType=function-call  IsSimulinkFunction=on  FunctionName=MagnMeasurementFcn_RIEKF  VariantControl=Variant
  Add : Sum
  Data Type Conversion1 : DataTypeConversion  OutDataTypeStr=single  SaturateOnIntegerOverflow=off  RndMeth=Floor
  MATLAB Function : MATLAB Function  TreatAsAtomicUnit=on
  Product : Product  Multiplication=Matrix(*)
  Selector : Selector  InputPortWidth=state_dim  IndexOptions=Index vector (dialog)  Indices=[1 2 3]  OutputSizes=1
  x : ArgIn  DisableCoverage=on  OutDataTypeStr=single  PortDimensions=state_dim  ArgumentName=x
  v : ArgIn  DisableCoverage=on  Port=2  OutDataTypeStr=single  PortDimensions=3  ArgumentName=v
  y : ArgOut  DisableCoverage=on  OutDataTypeStr=single  PortDimensions=3  ArgumentName=y
  wires:
  Selector/1 -> MATLAB Function/3(dtheta)
  xstate/1 -> Selector/1
  Rbn/1 -> MATLAB Function/1(Rbn)
  Data Type Conversion1/1 -> Product/1
  v/1 -> Add/2
  x/1 -> Product/2
  Magn/1 -> MATLAB Function/2(Magn)
  Add/1 -> y/1
  Product/1 -> Add/1
  MATLAB Function/1(H) -> Data Type Conversion1/1

== system VB_RI_EKF_GNSS_INS25/ISUS_RIEKF3/Error State Kalman Filter M3/Simulink Function - GPS Measurements3 ==
  Rbn : Inport
  vn : Inport  Port=2
  Rab : Inport  Port=3
  vel_wind_NED : Inport  Port=4
  AirspeedMeasurementFcn_RIEKF : TriggerPort  TriggerType=function-call  IsSimulinkFunction=on  FunctionName=AirspeedMeasurementFcn_RIEKF  VariantControl=Variant
  Add : Sum
  Data Type Conversion1 : DataTypeConversion  OutDataTypeStr=single  SaturateOnIntegerOverflow=off  RndMeth=Floor
  MATLAB Function : MATLAB Function  TreatAsAtomicUnit=on
  Product : Product  Multiplication=Matrix(*)
  x : ArgIn  DisableCoverage=on  OutDataTypeStr=single  PortDimensions=state_dim  ArgumentName=x
  v : ArgIn  DisableCoverage=on  Port=2  OutDataTypeStr=single  PortDimensions=3  ArgumentName=v
  y : ArgOut  DisableCoverage=on  OutDataTypeStr=single  PortDimensions=3  ArgumentName=y
  wires:
  vel_wind_NED/1 -> MATLAB Function/4(v_wind)
  Rab/1 -> MATLAB Function/2(Rab)
  vn/1 -> MATLAB Function/3(vn)
  Rbn/1 -> MATLAB Function/1(Rbn)
  Data Type Conversion1/1 -> Product/1
  v/1 -> Add/2
  x/1 -> Product/2
  Add/1 -> y/1
  Product/1 -> Add/1
  MATLAB Function/1(H) -> Data Type Conversion1/1

== system VB_RI_EKF_GNSS_INS25/ISUS_RIEKF3/Error State Kalman Filter M3/Simulink Function - State Transition ==
  DCM_b_n : Inport
  vn : Inport  Port=2  PortDimensions=[3,1]
  pn : Inport  Port=3  PortDimensions=[3,1]
  stateTransitionFcn_RIEKF : TriggerPort  TriggerType=function-call  IsSimulinkFunction=on  FunctionName=stateTransitionFcn_RIEKF  FunctionVisibility=scoped  VariantControl=Variant
  Add : Sum
  Cal Phi : Subsystem
  Constant : Constant  Value=dt  OutDataTypeStr=single
  Data Type Conversion1 : DataTypeConversion  OutDataTypeStr=single  SaturateOnIntegerOverflow=off  RndMeth=Floor
  Data Type Conversion6 : DataTypeConversion  OutDataTypeStr=single  SaturateOnIntegerOverflow=off  RndMeth=Floor
  MATLAB Function : MATLAB Function  TreatAsAtomicUnit=on
  Product1 : Product  Multiplication=Matrix(*)
  Product2 : Product  Multiplication=Matrix(*)
  x : ArgIn  DisableCoverage=on  OutDataTypeStr=single  PortDimensions=state_dim  ArgumentName=x
  w : ArgIn  Port=2  OutDataTypeStr=single  PortDimensions=cov_dim  ArgumentName=w
  xNext : ArgOut  DisableCoverage=on  OutDataTypeStr=single  PortDimensions=state_dim  ArgumentName=xNext
  wires:
  Data Type Conversion1/1 -> Add/1
  pn/1 -> Cal Phi/3(pn), MATLAB Function/3(pn)
  vn/1 -> Cal Phi/2(vn), MATLAB Function/2(vn)
  [DCM_b_n] -> Cal Phi/1(Rbn)
  Data Type Conversion6/1 -> Add/2
  Cal Phi/1(Phi) -> Product2/1
  DCM_b_n/1 -> [DCM_b_n]
  Constant/1 -> MATLAB Function/4(dt)
  [DCM_b_n] -> MATLAB Function/1(Rbn)
  Add/1 -> xNext/1
  Product1/1 -> Data Type Conversion1/1
  w/1 -> Product1/2
  MATLAB Function/1(G) -> Product1/1
  Product2/1 -> Data Type Conversion6/1
  x/1 -> Product2/2

== system VB_RI_EKF_GNSS_INS25/ISUS_RIEKF3/Error State Kalman Filter M3/Simulink Function - State Transition1 ==
  DCM_b_n : Inport
  vn : Inport  Port=2  PortDimensions=[3,1]
  pn : Inport  Port=3  PortDimensions=[3,1]
  stateFcn_RIEKFJacobian : TriggerPort  TriggerType=function-call  IsSimulinkFunction=on  FunctionName=stateFcn_RIEKFJacobian  FunctionVisibility=scoped  VariantControl=Variant
  Cal Phi : Subsystem
  Constant : Constant  Value=dt  OutDataTypeStr=single
  Data Type Conversion1 : DataTypeConversion  OutDataTypeStr=single  SaturateOnIntegerOverflow=off  RndMeth=Floor
  Data Type Conversion6 : DataTypeConversion  OutDataTypeStr=single  SaturateOnIntegerOverflow=off  RndMeth=Floor
  MATLAB Function : MATLAB Function  TreatAsAtomicUnit=on
  Terminator : Terminator
  Terminator1 : Terminator
  x : ArgIn  DisableCoverage=on  OutDataTypeStr=single  PortDimensions=state_dim  ArgumentName=x
  w : ArgIn  Port=2  OutDataTypeStr=single  PortDimensions=cov_dim  ArgumentName=w
  A : ArgOut  DisableCoverage=on  OutDataTypeStr=single  PortDimensions=[state_dim,state_dim]  ArgumentName=A
  G : ArgOut  Port=2  OutDataTypeStr=single  PortDimensions=[15,12]  ArgumentName=G
  wires:
  Data Type Conversion1/1 -> A/1
  Data Type Conversion6/1 -> G/1
  Cal Phi/1(Phi) -> Data Type Conversion1/1
  MATLAB Function/1(G) -> Data Type Conversion6/1
  x/1 -> Terminator1/1
  w/1 -> Terminator/1
  [DCM_b_n] -> MATLAB Function/1(Rbn)
  Constant/1 -> MATLAB Function/4(dt)
  DCM_b_n/1 -> [DCM_b_n]
  [DCM_b_n] -> Cal Phi/1(Rbn)
  vn/1 -> MATLAB Function/2(vn), Cal Phi/2(vn)
  pn/1 -> MATLAB Function/3(pn), Cal Phi/3(pn)

== system VB_RI_EKF_GNSS_INS25/ISUS_RIEKF3/Error State Kalman Filter M3/Subsystem ==
  data : Inport
  Detect Change : simulink/Logic and Bit Operations/Detect Change  vinit=0  InputProcessing=Columns as channels (frame based)  OutDataTypeStr=boolean
  Selector : Selector  InputPortWidth=3  IndexOptions=Index vector (dialog)  Indices=[3]  OutputSizes=1
  Zero-Order Hold : ZeroOrderHold  SampleTime=0.2
  Zero-Order Hold1 : ZeroOrderHold  SampleTime=0.01
  flag : Outport
  wires:
  Zero-Order Hold/1 -> Selector/1
  data/1 -> Zero-Order Hold/1
  Selector/1 -> Zero-Order Hold1/1
  Detect Change/1 -> flag/1
  Zero-Order Hold1/1 -> Detect Change/1

== system VB_RI_EKF_GNSS_INS25/ISUS_RIEKF3/Error State Kalman Filter M3/Subsystem1 ==
  v_I : Inport
  v_G : Inport  Port=2
  p_I : Inport  Port=3
  p_G : Inport  Port=4
  Enable : EnablePort
  Add1 : Sum  Inputs=+-
  Add2 : Sum  Inputs=+-
  Data Type Conversion : DataTypeConversion  OutDataTypeStr=single  SaturateOnIntegerOverflow=off  RndMeth=Floor
  Data Type Conversion2 : DataTypeConversion  OutDataTypeStr=single  SaturateOnIntegerOverflow=off  RndMeth=Floor
  Gain : Gain  Gain=-1
  Mux2 : Mux  Inputs=2
  dv/dp : Outport
  wires:
  p_G/1 -> Add1/2
  Gain/1 -> dv/dp/1
  v_I/1 -> Add2/1
  Add2/1 -> Data Type Conversion2/1
  Add1/1 -> Data Type Conversion/1
  p_I/1 -> Add1/1
  Data Type Conversion/1 -> Mux2/2
  v_G/1 -> Add2/2
  Data Type Conversion2/1 -> Mux2/1
  Mux2/1 -> Gain/1

== system VB_RI_EKF_GNSS_INS25/ISUS_RIEKF3/Error State Kalman Filter M3/Subsystem3 ==
  data : Inport
  Detect Change : simulink/Logic and Bit Operations/Detect Change  vinit=0  InputProcessing=Columns as channels (frame based)  OutDataTypeStr=boolean
  From Workspace1 : FromWorkspace  Commented=on  VariableName=[All.t',All.vn]
  From Workspace2 : FromWorkspace  VariableName=[time(1:(end-1)),FCS1.data_hf_st.lat(1:(end-1))]
  Selector : Selector  InputPortWidth=3  IndexOptions=Index vector (dialog)  Indices=[3]  OutputSizes=1
  flag : Outport
  wires:
  From Workspace2/1 -> Detect Change/1  "lat"
  data/1 -> Selector/1
  Detect Change/1 -> flag/1

== system VB_RI_EKF_GNSS_INS25/ISUS_RIEKF3/Error State Kalman Filter M3/bak ==
  From1 : From  Commented=on  GotoTag=wxyz
  From11 : From  Commented=on  GotoTag=p_INS
  From14 : From  Commented=on  GotoTag=DCM_b_n
  From2 : From  Commented=on  GotoTag=fbxyz
  From3 : From  Commented=on  GotoTag=ZUPTenable
  From4 : From  Commented=on  GotoTag=v_INS
  From5 : From  Commented=on  GotoTag=fex
  From6 : From  Commented=on  GotoTag=DCM_b_n
  From9 : From  Commented=on  GotoTag=DCM_b_n
  Goto6 : Goto  Commented=on  GotoTag=ZUPTenable
  MATLAB Function1 : MATLAB Function  Commented=on  TreatAsAtomicUnit=on
  Memory1 : Memory  Commented=on
  RIEKF : MATLAB Function  Commented=on  TreatAsAtomicUnit=on
  Rate Transition2 : RateTransition  Commented=on  OutPortSampleTime=dt
  Scope10 : Scope  Commented=on  NumInputPorts=2
  Simulink Function - GPS Measurements1 : Subsystem  Commented=on  TreatAsAtomicUnit=on
  Simulink Function - GPS Measurements2 : Subsystem  Commented=on  TreatAsAtomicUnit=on
  Simulink Function - State Transition Jacobian : Subsystem  Commented=on  TreatAsAtomicUnit=on
  Unscented Kalman Filter1 : sharedTrackingLibrary/Unscented Kalman Filter  Commented=on  StateTransitionFcn=stateTransitionFcn_Dyn  HasAdditiveProcessNoise=Nonadditive  ProcessNoise=1  HasTimeVaryingProcessNoise=on  HasStateTransitionFcnExtraArgument=0  InitialState=zeros(18,1)  InitialStateCovariance=diag([1*ones(3,1);0.1*ones(3,1);0.001*ones(3,1);0.001*ones(6,1);0.1*ones(3,1)]);  Alpha=1e-2  Beta=2  Kappa=0  MeasurementFcn1=GPSMeasurementFcn_Dyn  HasMeasurementEnablePort1=on  HasAdditiveMeasurementNoise1=Nonadditive  MeasurementNoise1=1  HasTimeVaryingMeasurementNoise1=on  HasMeasurementFcnExtraArgument1=0  HasMeasurementWrapping1=off  MeasurementFcn2=DynamicMeasurementFcn_Dyn  HasMeasurementEnablePort2=on  HasAdditiveMeasurementNoise2=Nonadditive  MeasurementNoise2=1  HasTimeVaryingMeasurementNoise2=on  HasMeasurementFcnExtraArgument2=0  HasMeasurementWrapping2=off  MeasurementFcn3=myMeasurementFcn  HasMeasurementEnablePort3=off  HasAdditiveMeasurementNoise3=Additive  MeasurementNoise3=1  HasTimeVaryingMeasurementNoise3=off  HasMeasurementFcnExtraArgument3=0  HasMeasurementWrapping3=off  MeasurementFcn4=myMeasurementFcn  HasMeasurementEnablePort4=off  HasAdditiveMeasurementNoise4=Additive  MeasurementNoise4=1  HasTimeVaryingMeasurementNoise4=off  HasMeasurementFcnExtraArgument4=0  HasMeasurementWrapping4=off  MeasurementFcn5=myMeasurementFcn  HasMeasurementEnablePort5=off  HasAdditiveMeasurementNoise5=Additive  MeasurementNoise5=1  HasTimeVaryingMeasurementNoise5=off  HasMeasurementFcnExtraArgument5=0  HasMeasurementWrapping5=off  EnableMultirate=off  StateTransitionFcnSampleTime=1  MeasurementFcn1SampleTime=1  MeasurementFcn2SampleTime=1  MeasurementFcn3SampleTime=1  MeasurementFcn4SampleTime=1  MeasurementFcn5SampleTime=1  UseCurrentEstimator=on  OutputStateCovariance=on  DataType=single  SampleTime=0.01  NumberOfMeasurements=2
  Out1 : Outport
  wires:
  From14/1 -> Simulink Function - GPS Measurements1/1(DCM_b_n)
  From4/1 -> Simulink Function - State Transition Jacobian/2(vn)
  From9/1 -> Simulink Function - State Transition Jacobian/1(DCM_b_n)
  From11/1 -> Simulink Function - State Transition Jacobian/3(pn)
  From3/1 -> Rate Transition2/1
  MATLAB Function1/2(ZeroVelDetectFlagold) -> Scope10/2
  From6/1 -> MATLAB Function1/1(Cbn)
  From2/1 -> MATLAB Function1/3(fbxyz)
  From5/1 -> Memory1/1
  MATLAB Function1/1(ZeroVelDetectFlag) -> Goto6/1, Scope10/1
  From1/1 -> MATLAB Function1/2(wxyz)
  Rate Transition2/1 -> Out1/1
  Memory1/1 -> MATLAB Function1/4(fex)

== system VB_RI_EKF_GNSS_INS25/ISUS_RIEKF3/INS propogation/Init_PVQ ==
  QGC_sensor_reinit : Inport
  accl_B_m/s2_LPF : Inport  Port=2
  Magn_B_guess_LPF : Inport  Port=3
  pos_NED : Inport  Port=4
  vel_NED : Inport  Port=5
  Add : Sum
  Add1 : Sum
  Constant1 : Constant  OutDataTypeStr=uint8
  Constant2 : Constant  Value=[0;0;0]  OutDataTypeStr=single
  Constant3 : Constant  Value=[0;0;0]  OutDataTypeStr=single
  Constant4 : Constant  Value=[vn0;ve0;vd0]  OutDataTypeStr=single
  Constant5 : Constant  Value=[pn0;pe0;pd0]  OutDataTypeStr=single
  Detect Increase : simulink/Logic and Bit Operations/Detect Increase  vinit=0.0  OutDataTypeStr=boolean
  Horizontal_attitude : Subsystem  TreatAsAtomicUnit=on
  Memory : Memory
  Scope : Scope  NumInputPorts=2
  Scope1 : Scope
  Subsystem : Subsystem
  Subsystem1 : Subsystem
  Subsystem2 : Subsystem
  Switch{,1..3} (4 alike) : Switch  Criteria=u2 > Threshold  SaturateOnIntegerOverflow=off  InputSameDT=off
  quat_0 : Outport
  v0 : Outport  Port=2
  p0 : Outport  Port=3
  wires:
  pos_NED/1 -> Add1/1
  Constant5/1 -> Add1/2
  Constant4/1 -> Add/2
  vel_NED/1 -> Add/1
  Switch/1 -> quat_0/1
  Subsystem1/1(mean_data) -> Horizontal_attitude/2(Magn_mean_B_guess_LPF)
  Subsystem/1(mean_data) -> Horizontal_attitude/1(accl_mean_B_m/s_LPF)
  Memory/1 -> Switch1/3
  Subsystem2/1(Quat0) -> Switch/3
  Horizontal_attitude/1(quat_0) -> Switch/1
  Constant1/1 -> Switch1/1
  Switch1/1 -> Memory/1, Switch2/2, Switch3/2, Switch/2, Scope1/1
  accl_B_m/s2_LPF/1 -> Subsystem/1(data)
  QGC_sensor_reinit/1 -> Detect Increase/1, Scope/1
  Magn_B_guess_LPF/1 -> Subsystem1/1(data)
  Detect Increase/1 -> Horizontal_attitude/Enable, Switch1/2, Scope/2
  Constant2/1 -> Switch2/3
  Constant3/1 -> Switch3/3
  Switch2/1 -> v0/1
  Switch3/1 -> p0/1
  Add1/1 -> Switch3/1
  Add/1 -> Switch2/1

== system VB_RI_EKF_GNSS_INS25/ISUS_RIEKF3/INS propogation/accl bias compensation ==
  QGC_init : Inport
  raw <accl_B_m/s2_LPF> : Inport  Port=2
  dda : Inport  Port=3
  Add2 : Sum
  Data Type Conversion6 : DataTypeConversion  OutDataTypeStr=single  SaturateOnIntegerOverflow=off  RndMeth=Floor
  error compensation1 : Subsystem
  fb : Outport  PortDimensions=3
  da : Outport  Port=2  PortDimensions=3
  wires:
  QGC_init/1 -> error compensation1/2(QGC_init)
  error compensation1/1(da) -> da/1, Add2/2
  Add2/1 -> Data Type Conversion6/1
  Data Type Conversion6/1 -> fb/1
  raw <accl_B_m/s2_LPF>/1 -> Add2/1
  dda/1 -> error compensation1/1(dda)
